simulink library "Enthalpy2Temperature"  (Simulink 8.2)
settings: Solver=ode45  StartTime=0.0  StopTime=10.0  RelTol=1e-3
undefined symbols (not defined in the file): CarnotCallbacks_Enthalpy2Temperature
settings Model: Creator=lena.frank  LastModifiedBy=drhf

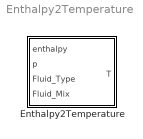
== system Enthalpy2Temperature ==
  Enthalpy2Temperature : Subsystem  LoadFcn=CarnotCallbacks_Enthalpy2Temperature('LoadFcn');  VariantControl=CarlibClassic  mask(Enthalpy to Temperature){DEBUGLEVEL=WARNINGLEVEL, MAXTOTALMESSAGES=inf, MAXCONSECUTIVEMESSAGES=inf, WRITETOFILE=0, FILENAME='errors.txt'}
      mask prompts: DEBUGLEVEL "Debug level"; MAXTOTALMESSAGES "maximum number of total warning"; MAXCONSECUTIVEMESSAGES "maximum number of consecutive warnings"; WRITETOFILE "write messages to file"; FILENAME "filename for error messages"
      mask help:
      | Calculates the temperature  [°C] from the fluid Enthalpy [J/kg].
      | Enthalpy may be a scalar or a vector. All other inputs must be scalar.
      | FluidType        Remarks
      | 1: water          fluid mix is vapourcontent in the 2-phase region
      | 2: air              fluid mix is (kg water) / (kg dry air)
      | 3: cotton oil       -
      | 4: silicone oil     -
      | 5: water-glycol   fluid mix is volume partition [0..1] of propylen glycol
      | 6: Tyfocor LS     function only available in liquid phase
      | 7: Water Constant - function not defined
      | 8: Air Constant - function not defined
      mask init:
      | %global debug level
      | [DEBUGLEVEL, MAXTOTALMESSAGES, MAXCONSECUTIVEMESSAGES, WRITETOFILE, FILENAME] = CarnotCallbacks_Enthalpy2Temperature('CheckDebugLevels', DEBUGLEVEL, MAXTOTALMESSAGES, MAXCONSECUTIVEMESSAGES, WRITETOFILE, FILENAME);
      mask Help: web(fullfile(path_carnot('help'),'enthalpy2temperature.html'),'-helpbrowser')
      mask TypeOptions DEBUGLEVEL: DEBUGLEVEL | INFOLEVEL | WARNINGLEVEL | ERRORLEVEL | FATALLEVEL | NOLEVEL
      mask DialogControl ParameterTabVar0 Prompt: Debugging

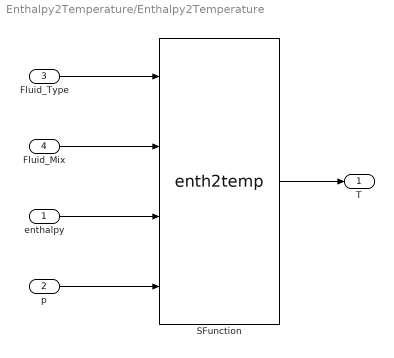
== system Enthalpy2Temperature/Enthalpy2Temperature ==
  enthalpy : Inport
  p : Inport  Port=2
  Fluid_Type : Inport  Port=3
  Fluid_Mix : Inport  Port=4
  SFunction : S-Function  FunctionName=enth2temp  Parameters=DEBUGLEVEL,MAXTOTALMESSAGES,MAXCONSECUTIVEMESSAGES,WRITETOFILE,FILENAME  EnableBusSupport=off
  T : Outport
  wires:
  p/1 -> SFunction/4
  enthalpy/1 -> SFunction/3
  Fluid_Mix/1 -> SFunction/2
  Fluid_Type/1 -> SFunction/1
  SFunction/1 -> T/1
